simulink model "Custom_Calib_Host"  (R2025b)
settings: Solver=VariableStepAuto  StartTime=0.0  StopTime=inf  RelTol=1e-3
libraries: instrumentseriallib x3

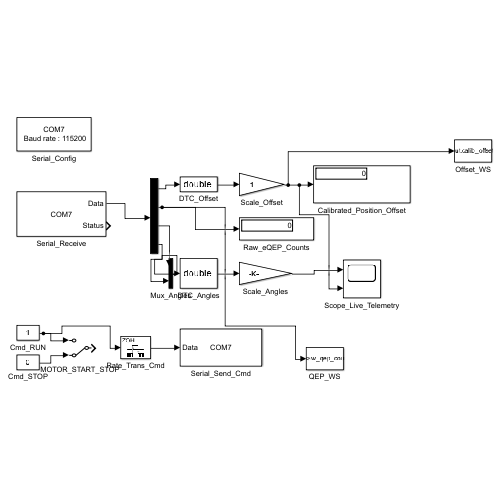
[thumbnail: Simulink's stored preview of the top-level diagram]
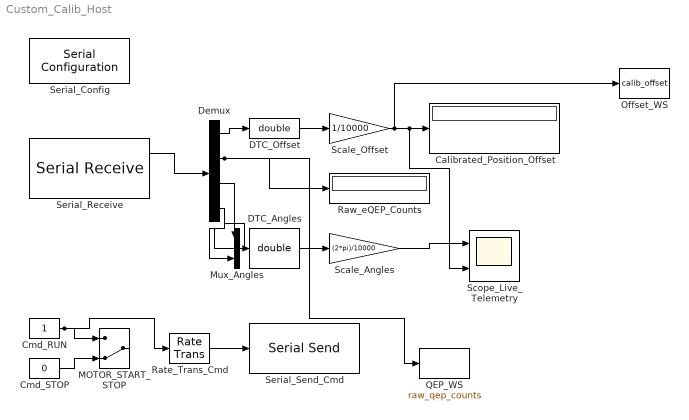
== system Custom_Calib_Host ==
  Calibrated_Position_Offset : Display
  Cmd_RUN : Constant  OutDataTypeStr=uint8
  Cmd_STOP : Constant  Value=0  OutDataTypeStr=uint8
  DTC_Angles : DataTypeConversion  OutDataTypeStr=double  SaturateOnIntegerOverflow=off  RndMeth=Floor
  DTC_Offset : DataTypeConversion  OutDataTypeStr=double  SaturateOnIntegerOverflow=off  RndMeth=Floor
  Demux : Demux
  MOTOR_START_STOP : ManualSwitch  CurrentSetting=0
  Mux_Angles : Mux  Inputs=2
  Offset_WS : ToWorkspace  VariableName=calib_offset  SaveFormat=Structure With Time  SampleTime=-1
  QEP_WS : ToWorkspace  VariableName=raw_qep_counts  SaveFormat=Structure With Time  SampleTime=-1
  Rate_Trans_Cmd : RateTransition  OutPortSampleTime=0.05
  Raw_eQEP_Counts : Display
  Scale_Angles : Gain  Gain=(2*pi)/10000
  Scale_Offset : Gain  Gain=1/10000
  Scope_Live_Telemetry : Scope  NumInputPorts=2
  Serial_Config : instrumentseriallib/Serial Configuration  Priority=-200000  PortSel=COM7  Port=COM7  ComPort=COM7  BaudRate=115200  DataBits=8  Parity=none  StopBits=1  ByteOrder=little-endian  FlowControl=none  Timeout=10  SimulateUsing=Interpreted execution  BlockInModel=on  aMode=1
  Serial_Receive : instrumentseriallib/Serial Receive  Priority=1  PortSel=COM7  Port=COM7  ComPort=COM7  DataType=uint16  SaveDataType=uint8  ToggleHeader=on  Header='SS'  ToggleDataSize=on  DataSize=[4 1]  ToggleTerminator=off  Terminator=<none>  CustomTerminator=[]  InputFormat=Column major  EnableBlockingMode=off  ActionDataUnavailable=Output last received value  ActionWhenDataUnavailable=Output last received value  CustomValue=0  SampleTime=0.01  SimulateUsing=Interpreted execution  BlockInModel=on  aMode=1  LibraryInUse=instrumentlib
  Serial_Send_Cmd : instrumentseriallib/Serial Send  Priority=1  PortSel=COM7  Port=COM7  ComPort=COM7  Header=[83, 84]  Terminator=<none>  CustomTerminator=[]  EnableBlockingMode=off  SimulateUsing=Interpreted execution  BlockInModel=on  aMode=1
  wires:
  Serial_Receive/1 -> Demux/1
  Demux/1 -> DTC_Offset/1
  DTC_Offset/1 -> Scale_Offset/1
  Scale_Offset/1 -> Calibrated_Position_Offset/1, Scope_Live_Telemetry/2, Offset_WS/1
  Demux/2 -> Raw_eQEP_Counts/1, QEP_WS/1
  Demux/3 -> Mux_Angles/1
  Demux/4 -> Mux_Angles/2
  Mux_Angles/1 -> DTC_Angles/1
  DTC_Angles/1 -> Scale_Angles/1
  Scale_Angles/1 -> Scope_Live_Telemetry/1
  Cmd_RUN/1 -> MOTOR_START_STOP/1, Rate_Trans_Cmd/1
  Cmd_STOP/1 -> MOTOR_START_STOP/2
  Rate_Trans_Cmd/1 -> Serial_Send_Cmd/1
